simulink model "ired_toolbox"  (R2019b)
settings: Solver=VariableStepAuto  StartTime=0.0  StopTime=30  RelTol=1e-3
settings Model: Creator=srichard057  LastModifiedBy=srichard057

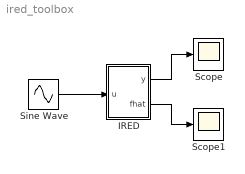
== system ired_toolbox ==
  IRED : Subsystem  InitFcn=|  mask{m=2, L=8, T=0.01, kappa=1.1, advanced=off, lambdai=0.5, R=0.01}
      | if str2double(get_param(gcb,'T')) == 0 || str2double(get_param(gcb,'L')) == 0
      |      
      |     error('L and T must be positive');
      |      
      | end
      mask prompts: m "Differentiation order m"; L "Lipschitz constant L for mth derivative"; T "Sampling time T"; kappa "Tuning parameter kappa > 1"; advanced "Enable advanced parametrization"; lambdai "Parameters [lambda_1 ... lambda_{m+1}]"; R "Tolerance of Newton-Raphson approximation R"
      mask init:
      | n = m+1;
      | 
      | 
      | % precompute C
      | C = zeros(n);
      | C(1,1) = 1;
      | for ii=2:n
      |     for jj=2:n
      |         C(ii,jj) = ((jj-2)*C(ii,jj-1)+(ii-1)*C(ii-1,jj-1))/(jj-1);
      |     end
      | end
      | TC = diag(T.^(0:-1:-(n-1)))*C;
      | Tn = T^n;
      mask Callback m:
      | %mask = Simulink.Mask.get(gcb);
      | lambdai = str2num(get_param(gcb,'lambdai'));
      | m = str2double(get_param(gcb, 'm'));
      | 
      | if strcmp(get_param(gcb, 'advanced'), 'on')
      |     lambdai = lambdai(:)';
      |     if length(lambdai) < m+1
      |         lambdan = lambdai(end);
      |         %lambdai = [lambdai(1:end-1) zeros(1,m+1-length(lambdai)) lambdan];
      |         lambdai = [zeros(1,m+1-length(lambdai)) lambdai];
      |     else
      |         %lambdai = [lambdai(1:m) lambdai(end)];
      |         lambdai = lambdai(length(lambdai)-m:end);
      |     end
      |     set_param(gcb, 'lambdai', mat2str(lambdai));
      | end
      | 
      | %mask.getParameter('lambdai').set('Value', mat2str(lambdai));
      mask Callback advanced:
      | mask = Simulink.Mask.get(gcb);
      | if strcmp(get_param(gcb, 'advanced'), 'on')
      |     variant =  'Choice';
      |     mask.getParameter('kappa').set('Enabled', 'off');
      |     mask.getParameter('lambdai').set('Visible', 'on');
      |     mask.getParameter('R').set('Visible', 'on');
      |     lambdai =str2num(get_param(gcb,'lambdai'));
      | 
      |     if strcmp(get_param(gcb, 'lambdai'), '0.5')
      |         kappa = str2double(get_param(gcb, 'kappa'));
      |         m = str2double(get_param(gcb, 'm'));
      |         lambdai = zeros(1,m+1);
      |         for ii=1:length(lambdai)
      |            lambdai(ii) = nchoosek(m+1,ii)*kappa^(ii/(m+1));
      |         end
      |         set_param(gcb, 'lambdai', mat2str(lambdai,5));
      |     end
      |     %lambdai = lambdai(:)';
      |     %if length(lambdai) < m+1
      |         %lambdai = [lambdai zeros(1,m+1-length(lambdai))];
      |     %else
      |         %lambdai = lambdai(1:m+1);
      |     %end
      |     %lambdai(end) = kappa;
      | 
      | else
      |     set_param(gcb, 'lambdai', '0.5');
      |     mask.getParameter('kappa').set('Enabled', 'on');
      |     mask.getParameter('lambdai').set('Visible', 'off');
      |     mask.getParameter('R').set('Visible', 'off');
      |     variant =  '(default)';
      | end
      | set_param(strcat(gcb, '/Differentiator Variants'), 'OverrideUsingVariant',variant);
      mask Callback lambdai:
      | if strcmp(get_param(gcb, 'advanced'), 'on')
      |     lambdai = str2num(get_param(gcb, 'lambdai'));
      |     set_param(gcb, 'kappa', mat2str(lambdai(end)));
      | end
  Scope : Scope
  Scope1 : Scope
  Sine Wave : Sin  Frequency=2  Phase=pi/2  SampleTime=0
  wires:
  Sine Wave/1 -> IRED/1(u)
  IRED/1(y) -> Scope/1
  IRED/2(fhat) -> Scope1/1

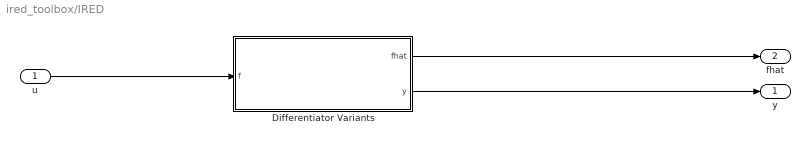
== system ired_toolbox/IRED ==
  u : Inport
  Differentiator Variants : Subsystem  VariantControlMode=Label  Variant=on  LabelModeActiveChoice=(default)
  y : Outport
  fhat : Outport  Port=2
  wires:
  u/1 -> Differentiator Variants/1(f)
  Differentiator Variants/2(y) -> y/1
  Differentiator Variants/1(fhat) -> fhat/1

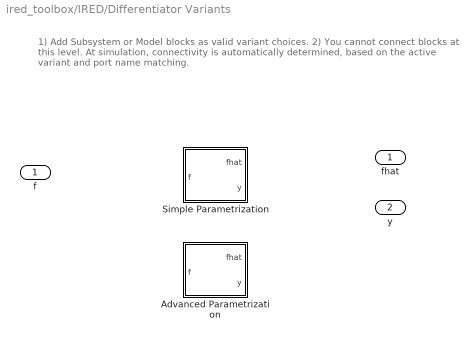
== system ired_toolbox/IRED/Differentiator Variants ==
  note: 1) Add Subsystem or Model blocks as valid variant choices.
      | 2) You cannot connect blocks at this level. At simulation, connectivity is automatically
      | determined, based on the active variant and port name matching.
  f : Inport
  Advanced Parametrization : Subsystem  VariantControl=Choice
  Simple Parametrization : Subsystem  VariantControl=(default)
  fhat : Outport
  y : Outport  Port=2

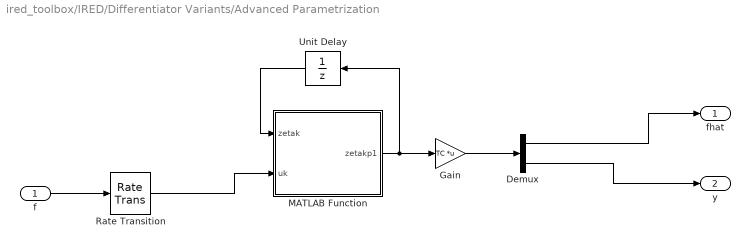
== system ired_toolbox/IRED/Differentiator Variants/Advanced Parametrization ==
  f : Inport
  Demux : Demux  Outputs=[1, n-1]
  Gain : Gain  Gain=TC  Multiplication=Matrix(K*u)
  MATLAB Function : MATLAB Function  TreatAsAtomicUnit=on
  Rate Transition : RateTransition  OutPortSampleTime=T
  Unit Delay : UnitDelay  InitialCondition=zeros(n,1)  SampleTime=-1  HasFrameUpgradeWarning=on
  fhat : Outport
  y : Outport  Port=2
  wires:
  Rate Transition/1 -> MATLAB Function/2(uk)
  Gain/1 -> Demux/1
  MATLAB Function/1(zetakp1) -> Gain/1, Unit Delay/1
  Unit Delay/1 -> MATLAB Function/1(zetak)
  Demux/2 -> y/1
  Demux/1 -> fhat/1
  f/1 -> Rate Transition/1

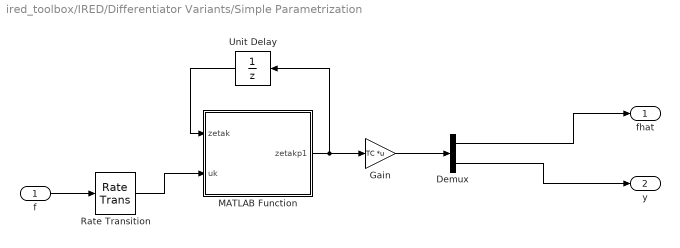
== system ired_toolbox/IRED/Differentiator Variants/Simple Parametrization ==
  f : Inport
  Demux : Demux  Outputs=[1, n-1]
  Gain : Gain  Gain=TC  Multiplication=Matrix(K*u)
  MATLAB Function : MATLAB Function  TreatAsAtomicUnit=on
  Rate Transition : RateTransition  OutPortSampleTime=T
  Unit Delay : UnitDelay  InitialCondition=zeros(n,1)  SampleTime=-1  HasFrameUpgradeWarning=on
  fhat : Outport
  y : Outport  Port=2
  wires:
  Rate Transition/1 -> MATLAB Function/2(uk)
  Demux/2 -> y/1
  Unit Delay/1 -> MATLAB Function/1(zetak)
  MATLAB Function/1(zetakp1) -> Unit Delay/1, Gain/1
  Gain/1 -> Demux/1
  f/1 -> Rate Transition/1
  Demux/1 -> fhat/1

== matlab function ired_toolbox/IRED/Differentiator Variants/Advanced Parametrization/MATLAB Function ==
  data: zetak input; zetakp1 output; uk input; L parameter; Tn parameter; n parameter; lambdai parameter; R parameter
function zetakp1 = diff_advanced(zetak, uk, L, Tn, n, lambdai, R)


zetakp1 = zeros(n,1);
bk = uk - sum(zetak);
LTn = L*Tn;
if abs(bk) > lambdai(end)*LTn
    beta = newton_root(bk, LTn, n, lambdai, R);
    zetakp1(n) = zetak(n) + lambdai(end)*LTn*sign(bk);
    for ii = (n-1):-1:1
        zetakp1(ii) = zetak(ii) + lambdai(ii)*LTn*beta^(n-ii)*sign(bk)+zetakp1(ii+1);
    end
else
    zetakp1(1) = uk;
    for ii=2:n
        zetakp1(ii) = zetakp1(ii-1)-zetak(ii-1);
    end
end


end

function beta = newton_root(bk, LTn, n,lambdai, R)

beta = (abs(bk)/LTn-lambdai(n))^(1/n);
epsilon = sum(beta.^(n-(1:n-1)).*lambdai(1:n-1));

while abs(epsilon) > R
    mu = n*beta^(n-1)+sum( (n-(1:n-1)).*lambdai(1:n-1).*beta.^(n-1-(1:n-1)));
    beta = beta - epsilon/mu;
    epsilon = beta^n-abs(bk)/LTn+sum(beta.^(n-(1:n)).*lambdai(1:n));
end


end

== matlab function ired_toolbox/IRED/Differentiator Variants/Simple Parametrization/MATLAB Function ==
  data: zetak input; zetakp1 output; uk input; L parameter; kappa parameter; Tn parameter; n parameter
function zetakp1 = diff_simple(zetak, uk, L, kappa, Tn, n)


%C = precompute_cij(n)
%Tn = T^n;
D = L*Tn*kappa;
zetakp1 = zeros(n,1);
bk = uk - sum(zetak);
if abs(bk) > D
    mu = (abs(bk)/D)^(1/n)-1;
    zetakp1(n) = zetak(n) + D*sign(bk);
    for ii = n-1:-1:1
        zetakp1(ii) = zetak(ii) + nchoosek(n,ii)*D*mu^(n-ii)*sign(bk)+zetakp1(ii+1);
    end
else
    zetakp1(1) = uk;
    for ii=2:n
        zetakp1(ii) = zetakp1(ii-1)-zetak(ii-1);
    end
end
